simulink model "encaout_lct"  (R2014a)
settings: Solver=FixedStepDiscrete  SolverMode=SingleTasking  StartTime=0.0  StopTime=10.0  RelTol=1e-3
settings Model: ExtModeTrigDuration=2  Creator=gcampa  LastModifiedBy=gcampa
settings OptimizationCC: OptimizeModelRefInitCode=on  LifeSpan=1
settings DebuggingCC: UnderspecifiedInitializationDetection=Classic  SolverPrmCheckMsg=none  FrameProcessingCompatibilityMsg=error  StateNameClashWarn=warning
settings HardwareCC: ProdBitPerInt=16  ProdBitPerPointer=8  ProdIntDivRoundTo=Zero  ProdEndianess=LittleEndian  ProdWordSize=8  ProdHWDeviceType=Atmel->AVR
settings RTWCC: SystemTargetFile=realtime.tlc  GenerateMakefile=off  TemplateMakefile=realtime.tmf  Description=Run on Target Hardware  RTWVerbose=off
settings STFCustomTargetCC: TargetLibSuffix=.a  GenerateSampleERTMain=on  ConcurrentExecutionCompliant=off  GeneratePreprocessorConditionals=Use local settings  ERTCustomFileBanners=on  SupportNonInlinedSFcns=off  SupportVariableSizeSignals=on  MATLABClassNameForMDSCustomization=Simulink.SoftwareTarget.ERTCustomization  GRTInterface=off  SystemTargetFile=realtime.tlc
settings ERTTargetCC: CombineOutputUpdateFcns=off  SupportContinuousTime=on  SupportVariableSizeSignals=on  ExtModeTransport=3  ExtModeMexFile=ext_serial_win32_comm  ExtModeMexArgs=0 1 9600  ERTSrcFileBannerTemplate=realtime_code_template.cgt  ERTHdrFileBannerTemplate=realtime_code_template.cgt  ERTDataSrcFileTemplate=realtime_code_template.cgt  ERTDataHdrFileTemplate=realtime_code_template.cgt  ERTCustomFileTemplate=realtime_file_process.tlc

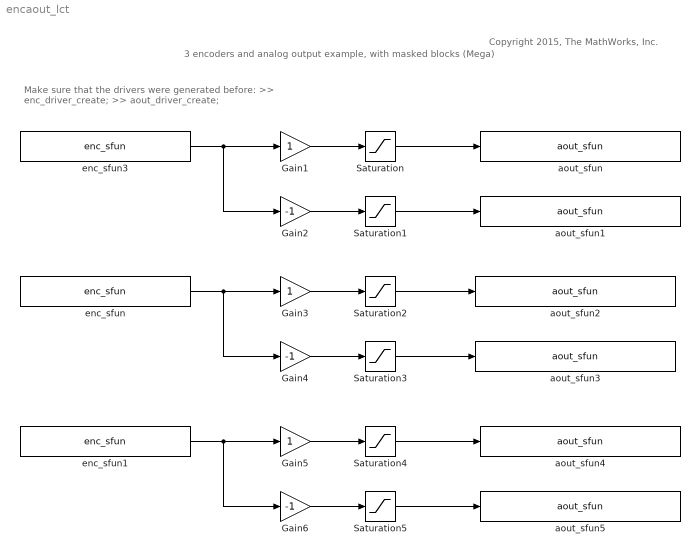
== system encaout_lct ==
  note: 3 encoders and analog output example, with masked blocks (Mega)
  note: Make sure that the drivers were generated before:
      | >> enc_driver_create;
      | >> aout_driver_create;
  note: Copyright 2015, The MathWorks, Inc.
  Gain1 : Gain  OutDataTypeStr=Inherit: Same as input
  Gain2 : Gain  Gain=-1  OutDataTypeStr=Inherit: Same as input
  Gain3 : Gain  OutDataTypeStr=Inherit: Same as input
  Gain4 : Gain  Gain=-1  OutDataTypeStr=Inherit: Same as input
  Gain5 : Gain  OutDataTypeStr=Inherit: Same as input
  Gain6 : Gain  Gain=-1  OutDataTypeStr=Inherit: Same as input
  Saturation{,1..5} (6 alike) : Saturate  UpperLimit=255  LowerLimit=0  OutDataTypeStr=Inherit: Inherit via back propagation
  aout_sfun : S-Function  FunctionName=aout_sfun  Parameters=SParameter1  mask(Legacy Function){SFunctionSpec=void aout_output(uint8 p1, uint8 u1), SParameter1=9, ShowSpec=on}
      mask prompts: SParameter1 "P1:"; ShowSpec "Display function specification"
      mask help:
      | This block allows you to call the legacy functions specified by the following Legacy Code Tool definition:
      | def.SFunctionName = 'aout_sfun';
      | def.OutputFcnSpec = 'void aout_output(uint8 p1, uint8 u1)';
      | def.StartFcnSpec = 'void aout_init(uint8 p1)';
      | def.HeaderFiles = {'aout_arduino.h'};
      | def.SourceFiles = {'Z:\28\mbelge.Bspkg15a.j198653\FX8\LCT\..\src\aout_arduino.cpp'};
      | def.IncPaths = {'Z:\28\mbelge.Bspkg15a.j198653\FX8\LCT\..\src'};
      mask Help: <p>This block was generated automatically by the Legacy Code Tool. For detailed help on this tool, call<a href="matlab:legacy_code('help')"> legacy_code('help')</a>.</p>
      mask Callback ShowSpec:
      | if strcmp(get_param(gcbh, 'ShowSpec'), 'on')
      |   set_param(gcbh, 'MaskDisplay', sprintf('fprintf(''%s'');', get_param(gcbh, 'SFunctionSpec')));
      | else
      |   set_param(gcbh, 'MaskDisplay', sprintf('fprintf(''%s'');', get_param(gcbh, 'FunctionName')));
      | end
      mask Display: fprintf('void aout_output(uint8 p1, uint8 u1)');
  aout_sfun1 : S-Function  FunctionName=aout_sfun  Parameters=SParameter1  mask(Legacy Function){SFunctionSpec=void aout_output(uint8 p1, uint8 u1), SParameter1=10, ShowSpec=on}
      mask prompts: SParameter1 "P1:"; ShowSpec "Display function specification"
      mask help:
      | This block allows you to call the legacy functions specified by the following Legacy Code Tool definition:
      | def.SFunctionName = 'aout_sfun';
      | def.OutputFcnSpec = 'void aout_output(uint8 p1, uint8 u1)';
      | def.StartFcnSpec = 'void aout_init(uint8 p1)';
      | def.HeaderFiles = {'aout_arduino.h'};
      | def.SourceFiles = {'Z:\28\mbelge.Bspkg15a.j198653\FX8\LCT\..\src\aout_arduino.cpp'};
      | def.IncPaths = {'Z:\28\mbelge.Bspkg15a.j198653\FX8\LCT\..\src'};
      mask Help: <p>This block was generated automatically by the Legacy Code Tool. For detailed help on this tool, call<a href="matlab:legacy_code('help')"> legacy_code('help')</a>.</p>
      mask Callback ShowSpec:
      | if strcmp(get_param(gcbh, 'ShowSpec'), 'on')
      |   set_param(gcbh, 'MaskDisplay', sprintf('fprintf(''%s'');', get_param(gcbh, 'SFunctionSpec')));
      | else
      |   set_param(gcbh, 'MaskDisplay', sprintf('fprintf(''%s'');', get_param(gcbh, 'FunctionName')));
      | end
      mask Display: fprintf('void aout_output(uint8 p1, uint8 u1)');
  aout_sfun2 : S-Function  FunctionName=aout_sfun  Parameters=SParameter1  mask(Legacy Function){SFunctionSpec=void aout_output(uint8 p1, uint8 u1), SParameter1=11, ShowSpec=on}
      mask prompts: SParameter1 "P1:"; ShowSpec "Display function specification"
      mask help:
      | This block allows you to call the legacy functions specified by the following Legacy Code Tool definition:
      | def.SFunctionName = 'aout_sfun';
      | def.OutputFcnSpec = 'void aout_output(uint8 p1, uint8 u1)';
      | def.StartFcnSpec = 'void aout_init(uint8 p1)';
      | def.HeaderFiles = {'aout_arduino.h'};
      | def.SourceFiles = {'Z:\28\mbelge.Bspkg15a.j198653\FX8\LCT\..\src\aout_arduino.cpp'};
      | def.IncPaths = {'Z:\28\mbelge.Bspkg15a.j198653\FX8\LCT\..\src'};
      mask Help: <p>This block was generated automatically by the Legacy Code Tool. For detailed help on this tool, call<a href="matlab:legacy_code('help')"> legacy_code('help')</a>.</p>
      mask Callback ShowSpec:
      | if strcmp(get_param(gcbh, 'ShowSpec'), 'on')
      |   set_param(gcbh, 'MaskDisplay', sprintf('fprintf(''%s'');', get_param(gcbh, 'SFunctionSpec')));
      | else
      |   set_param(gcbh, 'MaskDisplay', sprintf('fprintf(''%s'');', get_param(gcbh, 'FunctionName')));
      | end
      mask Display: fprintf('void aout_output(uint8 p1, uint8 u1)');
  aout_sfun3 : S-Function  FunctionName=aout_sfun  Parameters=SParameter1  mask(Legacy Function){SFunctionSpec=void aout_output(uint8 p1, uint8 u1), SParameter1=12, ShowSpec=on}
      mask prompts: SParameter1 "P1:"; ShowSpec "Display function specification"
      mask help:
      | This block allows you to call the legacy functions specified by the following Legacy Code Tool definition:
      | def.SFunctionName = 'aout_sfun';
      | def.OutputFcnSpec = 'void aout_output(uint8 p1, uint8 u1)';
      | def.StartFcnSpec = 'void aout_init(uint8 p1)';
      | def.HeaderFiles = {'aout_arduino.h'};
      | def.SourceFiles = {'Z:\28\mbelge.Bspkg15a.j198653\FX8\LCT\..\src\aout_arduino.cpp'};
      | def.IncPaths = {'Z:\28\mbelge.Bspkg15a.j198653\FX8\LCT\..\src'};
      mask Help: <p>This block was generated automatically by the Legacy Code Tool. For detailed help on this tool, call<a href="matlab:legacy_code('help')"> legacy_code('help')</a>.</p>
      mask Callback ShowSpec:
      | if strcmp(get_param(gcbh, 'ShowSpec'), 'on')
      |   set_param(gcbh, 'MaskDisplay', sprintf('fprintf(''%s'');', get_param(gcbh, 'SFunctionSpec')));
      | else
      |   set_param(gcbh, 'MaskDisplay', sprintf('fprintf(''%s'');', get_param(gcbh, 'FunctionName')));
      | end
      mask Display: fprintf('void aout_output(uint8 p1, uint8 u1)');
  aout_sfun4 : S-Function  FunctionName=aout_sfun  Parameters=SParameter1  mask(Legacy Function){SFunctionSpec=void aout_output(uint8 p1, uint8 u1), SParameter1=5, ShowSpec=on}
      mask prompts: SParameter1 "P1:"; ShowSpec "Display function specification"
      mask help:
      | This block allows you to call the legacy functions specified by the following Legacy Code Tool definition:
      | def.SFunctionName = 'aout_sfun';
      | def.OutputFcnSpec = 'void aout_output(uint8 p1, uint8 u1)';
      | def.StartFcnSpec = 'void aout_init(uint8 p1)';
      | def.HeaderFiles = {'aout_arduino.h'};
      | def.SourceFiles = {'Z:\28\mbelge.Bspkg15a.j198653\FX8\LCT\..\src\aout_arduino.cpp'};
      | def.IncPaths = {'Z:\28\mbelge.Bspkg15a.j198653\FX8\LCT\..\src'};
      mask Help: <p>This block was generated automatically by the Legacy Code Tool. For detailed help on this tool, call<a href="matlab:legacy_code('help')"> legacy_code('help')</a>.</p>
      mask Callback ShowSpec:
      | if strcmp(get_param(gcbh, 'ShowSpec'), 'on')
      |   set_param(gcbh, 'MaskDisplay', sprintf('fprintf(''%s'');', get_param(gcbh, 'SFunctionSpec')));
      | else
      |   set_param(gcbh, 'MaskDisplay', sprintf('fprintf(''%s'');', get_param(gcbh, 'FunctionName')));
      | end
      mask Display: fprintf('void aout_output(uint8 p1, uint8 u1)');
  aout_sfun5 : S-Function  FunctionName=aout_sfun  Parameters=SParameter1  mask(Legacy Function){SFunctionSpec=void aout_output(uint8 p1, uint8 u1), SParameter1=6, ShowSpec=on}
      mask prompts: SParameter1 "P1:"; ShowSpec "Display function specification"
      mask help:
      | This block allows you to call the legacy functions specified by the following Legacy Code Tool definition:
      | def.SFunctionName = 'aout_sfun';
      | def.OutputFcnSpec = 'void aout_output(uint8 p1, uint8 u1)';
      | def.StartFcnSpec = 'void aout_init(uint8 p1)';
      | def.HeaderFiles = {'aout_arduino.h'};
      | def.SourceFiles = {'Z:\28\mbelge.Bspkg15a.j198653\FX8\LCT\..\src\aout_arduino.cpp'};
      | def.IncPaths = {'Z:\28\mbelge.Bspkg15a.j198653\FX8\LCT\..\src'};
      mask Help: <p>This block was generated automatically by the Legacy Code Tool. For detailed help on this tool, call<a href="matlab:legacy_code('help')"> legacy_code('help')</a>.</p>
      mask Callback ShowSpec:
      | if strcmp(get_param(gcbh, 'ShowSpec'), 'on')
      |   set_param(gcbh, 'MaskDisplay', sprintf('fprintf(''%s'');', get_param(gcbh, 'SFunctionSpec')));
      | else
      |   set_param(gcbh, 'MaskDisplay', sprintf('fprintf(''%s'');', get_param(gcbh, 'FunctionName')));
      | end
      mask Display: fprintf('void aout_output(uint8 p1, uint8 u1)');
  enc_sfun : S-Function  FunctionName=enc_sfun  Parameters=SParameter1, SParameter2, SParameter3  mask(Legacy Function){SFunctionSpec=int16 y1 = enc_output(int16 p1), SParameter1=1, SParameter2=18, SParameter3=19, ShowSpec=on}
      mask prompts: SParameter1 "P1:"; SParameter2 "P2:"; SParameter3 "P3:"; ShowSpec "Display function specification"
      mask help:
      | This block allows you to call the legacy functions specified by the following Legacy Code Tool definition:
      | def.SFunctionName = 'enc_sfun';
      | def.OutputFcnSpec = 'int16 y1 = enc_output(int16 p1)';
      | def.StartFcnSpec = 'void enc_init(int16 p1, int16 p2, int16 p3)';
      | def.HeaderFiles = {'encoder_arduino.h'};
      | def.SourceFiles = {'Z:\28\mbelge.Bspkg15a.j198653\FX8\LCT\..\src\encoder_arduino.cpp'};
      | def.IncPaths = {'Z:\28\mbelge.Bspkg15a.j198653\FX8\LCT\..\src'};
      | def.SampleTime = 0.05;
      mask Help: <p>This block was generated automatically by the Legacy Code Tool. For detailed help on this tool, call<a href="matlab:legacy_code('help')"> legacy_code('help')</a>.</p>
      mask Callback ShowSpec:
      | if strcmp(get_param(gcbh, 'ShowSpec'), 'on')
      |   set_param(gcbh, 'MaskDisplay', sprintf('fprintf(''%s'');', get_param(gcbh, 'SFunctionSpec')));
      | else
      |   set_param(gcbh, 'MaskDisplay', sprintf('fprintf(''%s'');', get_param(gcbh, 'FunctionName')));
      | end
      mask Display: fprintf('int16 y1 = enc_output(int16 p1)');
  enc_sfun1 : S-Function  FunctionName=enc_sfun  Parameters=SParameter1, SParameter2, SParameter3  mask(Legacy Function){SFunctionSpec=int16 y1 = enc_output(int16 p1), SParameter1=2, SParameter2=20, SParameter3=21, ShowSpec=on}
      mask prompts: SParameter1 "P1:"; SParameter2 "P2:"; SParameter3 "P3:"; ShowSpec "Display function specification"
      mask help:
      | This block allows you to call the legacy functions specified by the following Legacy Code Tool definition:
      | def.SFunctionName = 'enc_sfun';
      | def.OutputFcnSpec = 'int16 y1 = enc_output(int16 p1)';
      | def.StartFcnSpec = 'void enc_init(int16 p1, int16 p2, int16 p3)';
      | def.HeaderFiles = {'encoder_arduino.h'};
      | def.SourceFiles = {'Z:\28\mbelge.Bspkg15a.j198653\FX8\LCT\..\src\encoder_arduino.cpp'};
      | def.IncPaths = {'Z:\28\mbelge.Bspkg15a.j198653\FX8\LCT\..\src'};
      | def.SampleTime = 0.05;
      mask Help: <p>This block was generated automatically by the Legacy Code Tool. For detailed help on this tool, call<a href="matlab:legacy_code('help')"> legacy_code('help')</a>.</p>
      mask Callback ShowSpec:
      | if strcmp(get_param(gcbh, 'ShowSpec'), 'on')
      |   set_param(gcbh, 'MaskDisplay', sprintf('fprintf(''%s'');', get_param(gcbh, 'SFunctionSpec')));
      | else
      |   set_param(gcbh, 'MaskDisplay', sprintf('fprintf(''%s'');', get_param(gcbh, 'FunctionName')));
      | end
      mask Display: fprintf('int16 y1 = enc_output(int16 p1)');
  enc_sfun3 : S-Function  FunctionName=enc_sfun  Parameters=SParameter1, SParameter2, SParameter3  mask(Legacy Function){SFunctionSpec=int16 y1 = enc_output(int16 p1), SParameter1=0, SParameter2=2, SParameter3=3, ShowSpec=on}
      mask prompts: SParameter1 "P1:"; SParameter2 "P2:"; SParameter3 "P3:"; ShowSpec "Display function specification"
      mask help:
      | This block allows you to call the legacy functions specified by the following Legacy Code Tool definition:
      | def.SFunctionName = 'enc_sfun';
      | def.OutputFcnSpec = 'int16 y1 = enc_output(int16 p1)';
      | def.StartFcnSpec = 'void enc_init(int16 p1, int16 p2, int16 p3)';
      | def.HeaderFiles = {'encoder_arduino.h'};
      | def.SourceFiles = {'Z:\28\mbelge.Bspkg15a.j198653\FX8\LCT\..\src\encoder_arduino.cpp'};
      | def.IncPaths = {'Z:\28\mbelge.Bspkg15a.j198653\FX8\LCT\..\src'};
      | def.SampleTime = 0.05;
      mask Help: <p>This block was generated automatically by the Legacy Code Tool. For detailed help on this tool, call<a href="matlab:legacy_code('help')"> legacy_code('help')</a>.</p>
      mask Callback ShowSpec:
      | if strcmp(get_param(gcbh, 'ShowSpec'), 'on')
      |   set_param(gcbh, 'MaskDisplay', sprintf('fprintf(''%s'');', get_param(gcbh, 'SFunctionSpec')));
      | else
      |   set_param(gcbh, 'MaskDisplay', sprintf('fprintf(''%s'');', get_param(gcbh, 'FunctionName')));
      | end
      mask Display: fprintf('int16 y1 = enc_output(int16 p1)');
  wires:
  Saturation/1 -> aout_sfun/1
  Gain1/1 -> Saturation/1
  enc_sfun3/1 -> Gain2/1, Gain1/1
  Gain2/1 -> Saturation1/1
  Saturation1/1 -> aout_sfun1/1
  Saturation2/1 -> aout_sfun2/1
  Gain3/1 -> Saturation2/1
  enc_sfun/1 -> Gain3/1, Gain4/1
  Gain4/1 -> Saturation3/1
  Saturation3/1 -> aout_sfun3/1
  Saturation4/1 -> aout_sfun4/1
  Gain5/1 -> Saturation4/1
  enc_sfun1/1 -> Gain6/1, Gain5/1
  Gain6/1 -> Saturation5/1
  Saturation5/1 -> aout_sfun5/1
